simulink model "DFIGAC"  (R2024a)
settings: Solver=ode23tb  StartTime=0.0  StopTime=10.0  RelTol=1e-4  AbsTol=1e-3
libraries: spsPowerPhasorLib x2, spsThreePhaseVIMeasurementLib x2, spsGroundLib x2, spsThreePhaseProgrammableVoltageSourceLib x1, spsThreePhaseParallelRLCLoadLib x1, spsThreePhaseTransformerTwoWindingsLib x1, spsWindTurbineDoublyFedInductionGeneratorPhasorTypeLib x1, sps_lib x1
settings Model: Creator=piyus  LastModifiedBy=piyus
settings SolverCC: SolverResetMethod=Robust

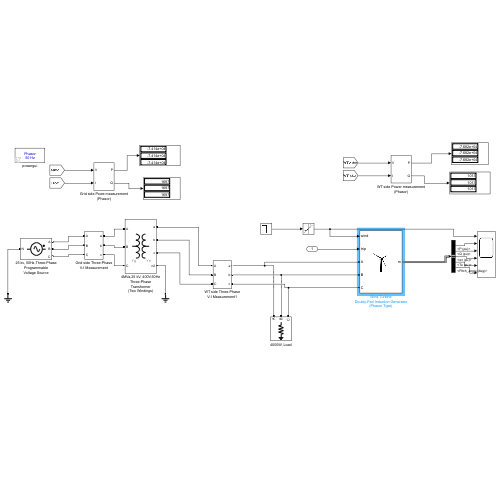
[thumbnail: Simulink's stored preview of the top-level diagram]
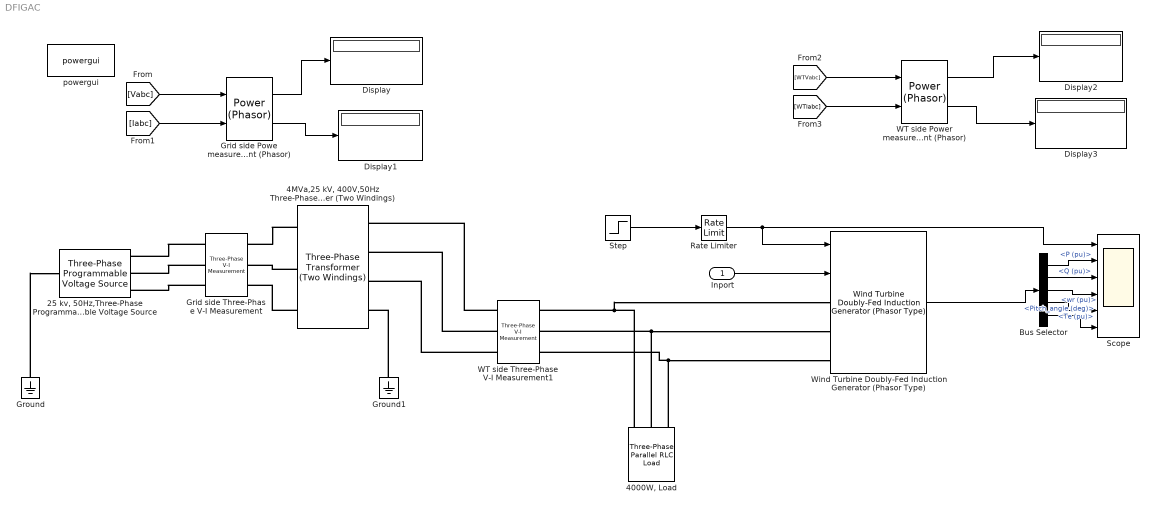
== system DFIGAC ==
  Inport : Inport
  "25 kv, 50Hz,Three-Phase Programmable Voltage Source" : spsThreePhaseProgrammableVoltageSourceLib/Three-Phase Programmable Voltage Source  PositiveSequence="[25e3  0 50]"  VariationEntity=None  VariationType=Table of time-amplitude pairs  VariationTypeAlt=Step  VariationStep=0.5  VariationRate=10  VariationMagnitude=0.3  VariationFrequency=2  VariationTiming=[1 2]  VariationPhaseA=off  Amplitudes=[1 0.8 1.2 1.0]  TimeValues=[0 0.1 0.15 0.2]  HarmonicGeneration=off  HarmonicA=[3 0.2 -25 0]  HarmonicB=[2 0.15 35 2]  Timing="[0.05  3]"  BusType=swing  Pref=0  Qref=0  Qmin=-inf  Qmax=inf
  "4000W, Load" : spsThreePhaseParallelRLCLoadLib/Three-Phase Parallel RLC Load  LConnTagsString=A|B|C  Configuration=Y (grounded)  NominalVoltage=400  Vabc=[1e3 1e3 1e3]  Vabcp=[1e3 1e3 1e3]  NominalFrequency=50  UnbalancedPower=off  ActivePower=4e3  InductivePower=0  CapacitivePower=0  Pabc=[10e3 9e3 11e3]  QLabc=[100 90 110]  QCabc=[100 90 110]  Pabcp=[10e3 9e3 11e3]  QLabcp=[100 90 110]  QCabcp=[100 90 110]  Measurements=None  LoadType=constant Z
  "4MVa,25 kV, 400V,50Hz Three-Phase Transformer (Two Windings)" : spsThreePhaseTransformerTwoWindingsLib/Three-Phase Transformer (Two Windings)  Winding1Connection=Yg  Winding2Connection=Yn  CoreType=Three single-phase transformers  SetSaturation=off  Hysteresis=off  DataFile='hysteresis'  SetInitialFlux=off  Measurements=None  UNITS=pu  NominalPower=[ 4e6 , 50 ]  Winding1=[ 25e3 , 0.002 , 0.08 ]  Winding2=[ 400 , 0.002 , 0.08 ]  Rm=500  Lm=inf  L0=0.5  Saturation=[ 0,0 ; 0.0024,1.2 ; 1.0,1.52 ]  InitialFluxes=[ 0.8 , -0.8 , 0.7 ]  BreakLoop=off  DiscreteSolver=Trapezoidal iterative  DataType=off  TransfoNumber=1
  Bus Selector : BusSelector  OutputSignals=P (pu),Q (pu),wr (pu),Te (pu),Pitch_angle (deg)
  Display{,1..3} (4 alike) : Display
  Grid side Powe measurement (Phasor) : spsPowerPhasorLib/Power (Phasor)
      settings: LibrarySourceBlock=|
      | sps_lib/Sensors and Measurements/Power
      | (Phasor)
  Grid side Three-Phase V-I Measurement : spsThreePhaseVIMeasurementLib/Three-Phase V-I Measurement  VoltageMeasurement=phase-to-ground  SetLabelV=on  LabelV=Vabc  Vpu=off  VpuLL=off  CurrentMeasurement=yes  SetLabelI=on  LabelI=Iabc  Ipu=off  Pbase=100e6  Vbase=500e3  OutputType=Complex  PhasorSimulation=on  PSBequivalent=0
  Ground : spsGroundLib/Ground  LConnTagsString=a
  Ground1 : spsGroundLib/Ground  LConnTagsString=a
  Rate Limiter : RateLimiter  RisingSlewLimit=10
  Scope : Scope  NumInputPorts=6
  Step : Step  Before=8  After=7  SampleTime=0
  WT side Power measurement (Phasor) : spsPowerPhasorLib/Power (Phasor)
      settings: LibrarySourceBlock=|
      | sps_lib/Sensors and Measurements/Power
      | (Phasor)
  WT side Three-Phase V-I Measurement1 : spsThreePhaseVIMeasurementLib/Three-Phase V-I Measurement  VoltageMeasurement=phase-to-ground  SetLabelV=on  LabelV=WTVabc  Vpu=off  VpuLL=off  CurrentMeasurement=yes  SetLabelI=on  LabelI=WTIabc  Ipu=off  Pbase=100e6  Vbase=500e3  OutputType=Complex  PhasorSimulation=on  PSBequivalent=0
  Wind Turbine Doubly-Fed Induction Generator (Phasor Type) : spsWindTurbineDoublyFedInductionGeneratorPhasorTypeLib/Wind Turbine Doubly-Fed Induction Generator (Phasor Type)  ExternalTm=off  nom=[1e6 400 50]  sta=[ 0.00706 0.171]  rot=[ 0.005 0.156]  Lm=2.90  mec=[5.04 0.01 3]  init=[0.2 0 0 0 0 0]  speed_power=[0 0; 0.24 0.007; 0.36 0.024; 0.6 0.112; 0.96 0.46; 1.2 0.898; 1.5 0.898]  Pmec=1e6  speed_ABCD=[0.7 0.71 1.2 1.21]  power_C=0.73  wind_point_C=10  pitch_gain=500  pitch_max=45  pitch_rate=2  Pmax=0.5  Lchoke=[0.15 0.15/100]  init_inductor=[0 90]  Vdc_nom=1000  capacitor=10000e-6  ControlVQ=Voltage regulation  Vref=1.0  ExternalVref=off  Qref=0  ExternalQref=off  Iq_ref=0  ExternalIqref=off  Kpi_volt_reg=[1.25 300]  Xs=0.02  Kpi_Q=[0.05 5]  Kpi_power_reg=[1 100]  Kpi_dc_reg=[0.002 0.05]  Kpi_grid_side_cur_reg=[1 100]  Kpi_rotor_side_cur_reg=[0.3 8]  V_slew_rate=100  Q_slew_rate=100  power_slew_rate=1  current_slew_rate=200
      settings: LibrarySourceBlock=|
      | sps_lib/Electrical Machines/Wind Turbine
      | Doubly-Fed Induction Generator
      | (Phasor Type)
  powergui : sps_lib/powergui  Priority=1  SimulationMode=Phasor  SampleTime=50e-6  frequency=50  Iterations=50  frequencyindice=50  Pbase=100e6  ErrMax=1e-4  UnitsV=kV  UnitsW=MW  buscounter=0  FunctionMessages=off  echomessages=off  EnableUseOfTLC=off  CurrentSourceSwitches=off  DisableSnubberDevices=off  DisableRonSwitches=off  DisableVfSwitches=off  DisplayEquations=off  AutomaticDiscreteSolvers=off  SolverType=Tustin/Backward Euler (TBE)  Interpol=off  ExternalGateDelay=off  methode=off  Ts=100  x0status=blocks  SPID=on  SwTol=0  HookPort=off  NonlinearTolerance=1e-4  nMaxIteration=100  ContinueOnMaxIteration=off  RestoreLinks=warning  ResistiveCurrentMeasurement=off  Frange=[0:2:500]  Ylog=off  Xlog=on  ShowGrid=off  save=off  variable=ZData  structure=0  ZoomFFT=off  StartTime=0.0  cycles=1  DisplayStyle=1  fundamental=60  FreqAxis=off  MaxFrequency=1000  frequencyindicesteady=1  RmsSteady=1  display=off
  wires:
  Step/1 -> Rate Limiter/1
  Rate Limiter/1 -> Wind Turbine Doubly-Fed Induction Generator (Phasor Type)/1, Scope/1
  Wind Turbine Doubly-Fed Induction Generator (Phasor Type)/1 -> Bus Selector/1
  Bus Selector/1 -> Scope/2  "<P (pu)>"
  Bus Selector/2 -> Scope/3  "<Q (pu)>"
  Bus Selector/3 -> Scope/4  "<wr (pu)>"
  Bus Selector/4 -> Scope/5  "<Te (pu)>"
  Bus Selector/5 -> Scope/6  "<Pitch_angle (deg)>"
  [Vabc] -> Grid side Powe measurement (Phasor)/1
  [Iabc] -> Grid side Powe measurement (Phasor)/2
  [WTVabc] -> WT side Power measurement (Phasor)/1
  [WTIabc] -> WT side Power measurement (Phasor)/2
  Grid side Powe measurement (Phasor)/2 -> Display1/1
  Grid side Powe measurement (Phasor)/1 -> Display/1
  WT side Power measurement (Phasor)/2 -> Display3/1
  Inport/1 -> Wind Turbine Doubly-Fed Induction Generator (Phasor Type)/2
  WT side Power measurement (Phasor)/1 -> Display2/1
  connections:
  Ground/LConn1 -- "25 kv, 50Hz,Three-Phase Programmable Voltage Source"/LConn1
  Grid side Three-Phase V-I Measurement/LConn1 -- "25 kv, 50Hz,Three-Phase Programmable Voltage Source"/RConn1
  Grid side Three-Phase V-I Measurement/LConn2 -- "25 kv, 50Hz,Three-Phase Programmable Voltage Source"/RConn2
  Grid side Three-Phase V-I Measurement/LConn3 -- "25 kv, 50Hz,Three-Phase Programmable Voltage Source"/RConn3
  "4MVa,25 kV, 400V,50Hz Three-Phase Transformer (Two Windings)"/LConn1 -- Grid side Three-Phase V-I Measurement/RConn1
  "4MVa,25 kV, 400V,50Hz Three-Phase Transformer (Two Windings)"/LConn2 -- Grid side Three-Phase V-I Measurement/RConn2
  "4MVa,25 kV, 400V,50Hz Three-Phase Transformer (Two Windings)"/LConn3 -- Grid side Three-Phase V-I Measurement/RConn3
  Ground1/LConn1 -- "4MVa,25 kV, 400V,50Hz Three-Phase Transformer (Two Windings)"/RConn4
  WT side Three-Phase V-I Measurement1/LConn1 -- "4MVa,25 kV, 400V,50Hz Three-Phase Transformer (Two Windings)"/RConn1
  WT side Three-Phase V-I Measurement1/LConn2 -- "4MVa,25 kV, 400V,50Hz Three-Phase Transformer (Two Windings)"/RConn2
  WT side Three-Phase V-I Measurement1/LConn3 -- "4MVa,25 kV, 400V,50Hz Three-Phase Transformer (Two Windings)"/RConn3
  "4000W, Load"/LConn1 -- Wind Turbine Doubly-Fed Induction Generator (Phasor Type)/LConn1 -- WT side Three-Phase V-I Measurement1/RConn1
  "4000W, Load"/LConn2 -- WT side Three-Phase V-I Measurement1/RConn2 -- Wind Turbine Doubly-Fed Induction Generator (Phasor Type)/LConn2
  "4000W, Load"/LConn3 -- WT side Three-Phase V-I Measurement1/RConn3 -- Wind Turbine Doubly-Fed Induction Generator (Phasor Type)/LConn3
